simulink model "tire"  (R2020b)
settings: Solver=VariableStepAuto  StartTime=0.0  StopTime=10.0  RelTol=1e-3
InitFcn:
  | mdl = 'tire';
  | wks = get_param(mdl, 'ModelWorkspace');
  | 
  | % ---- FRONT TIRES ----
  | 
  | % Load data for front tires
  | vals_struct_front = load('lateral_data_lut_FRONT.mat');
  | load_y_front = vals_struct_front.load_y;
  | 
  | % Set data for FR tire
  | sa_x_FR = vals_struct_front.sa_x;
  | lateral_coeff_FR = vals_struct_front.lat_coeff;
  | aligning_torque_FR = vals_struct_front.aligning_torque;
  | 
  | % Set data for FL tire
  | sa_x_FL = -flip(sa_x_FR);
  | lateral_coeff_FL = -flipud(lateral_coeff_FR);
  | aligning_torque_FL = -flipud(aligning_torque_FR);
  | 
  | % Set front workspace vars to this data
  | assignin(wks, 'sa_x_FR', sa_x_FR);
  | assignin(wks, 'sa_x_FL', sa_x_FL);
  | assignin(wks, 'load_y_front', load_y_front);
  | assignin(wks, 'lateral_coeff_FR', lateral_coeff_FR);
  | assignin(wks, 'lateral_coeff_FL', lateral_coeff_FL);
  | assignin(wks, 'aligning_torque_FR', aligning_torque_FR);
  | assignin(wks, 'aligning_torque_FL', aligning_torque_FL);
  | 
  | % ---- REAR TIRES ----
  | 
  | % Load data for rear tires
  | vals_struct_rear = load('lateral_data_lut_REAR.mat');
  | load_y_rear = vals_struct_rear.load_y;
  | 
  | % Set data for RR tire
  | sa_x_RR = vals_struct_rear.sa_x;
  | lateral_coeff_RR = vals_struct_rear.lat_coeff;
  | aligning_torque_RR = vals_struct_rear.aligning_torque;
  | 
  | % Set data for RL tire
  | sa_x_RL = -flip(sa_x_RR);
  | lateral_coeff_RL = -flipud(lateral_coeff_RR);
  | aligning_torque_RL = -flipud(aligning_torque_RR);
  | 
  | % Set rear workspace vars to this data
  | assignin(wks, 'sa_x_RR', sa_x_RR);
  | assignin(wks, 'sa_x_RL', sa_x_RL);
  | assignin(wks, 'load_y_rear', load_y_rear);
  | assignin(wks, 'lateral_coeff_RR', lateral_coeff_RR);
  | assignin(wks, 'lateral_coeff_RL', lateral_coeff_RL);
  | assignin(wks, 'aligning_torque_RR', aligning_torque_RR);
  | assignin(wks, 'aligning_torque_RL', aligning_torque_RL);
model workspace (MAT data in the model file):
  aligning_torque = []
  aligning_torque_FL = [0.632054514609 1.00030929496 1.3564832949 1.69993473408 2.03003955804 2.34619584294 2.64782835053 2.93439319713 3.20538259517 3.4603296206 3.69881295493 3.92046154611 ... (18361 elements, 301x61)]
  aligning_torque_FR = [-8.27629240449 -7.94698029872 -7.63155523092 -7.33058213037 -7.04459380991 -6.7740862219 -6.51951369497 -6.28128420344 -6.05975472552 -5.85522675004 -5.66794199447 -5.49807839857 ... (18361 elements, 301x61)]
  aligning_torque_RL = [53.8378936848 52.3526089047 50.876903499 49.4110361793 47.9552665479 46.509854779 45.0750612888 43.6511464002 42.23837 40.836991194 39.4472679592 38.069456796 ... (18361 elements, 301x61)]
  aligning_torque_RR = [57.9779733339 55.1587439621 52.2420091829 49.2227619878 46.0969933513 42.8622156405 39.5181440804 36.0675717001 32.5174763364 28.8803985882 25.1761245506 21.4336928492 ... (18361 elements, 301x61)]
  lateral_coeff = []
  lateral_coeff_FL = [-2.62522245811 -2.64027696786 -2.65519252593 -2.6699687689 -2.68460531112 -2.69910174378 -2.71345763408 -2.72767252434 -2.74174593098 -2.75567734364 -2.76946622413 -2.7831120054 ... (18361 elements, 301x61)]
  lateral_coeff_FR = [-2.31568506961 -2.3309279537 -2.34603248296 -2.3609983259 -2.37582512996 -2.39051252072 -2.40506010102 -2.41946745011 -2.43373412279 -2.44785964843 -2.46184353006 -2.47568524338 ... (18361 elements, 301x61)]
  lateral_coeff_RL = [-2.38815959379 -2.39206360714 -2.39593787741 -2.39978203345 -2.40359569234 -2.407378459 -2.41112992576 -2.4148496719 -2.41853726322 -2.42219225158 -2.42581417433 -2.42940255388 ... (18361 elements, 301x61)]
  lateral_coeff_RR = [-2.49073654046 -2.49455737452 -2.49834746536 -2.50210640915 -2.50583378914 -2.50952917523 -2.51319212352 -2.51682217581 -2.52041885907 -2.52398168491 -2.52751014907 -2.53100373076 ... (18361 elements, 301x61)]
  load_y = []
  load_y_front = [0 -20 -40 -60 -80 -100 -120 -140 -160 -180 -200 -220 -240 -260 -280 -300 -320 -340 -360 -380 -400 -420 -440 -460 -480 -500 -520 -540 -560 -580 -600 -620 -640 -660 -680 -700 -720 -740 -760 -780 -800 -820 -840 -860 -880 -900 -920 -940 -960 -980 -1000 -1020 -1040 -1060 -1080 -1100 -1120 -1140 -1160 -1180 -1200]
  load_y_rear = [0 -20 -40 -60 -80 -100 -120 -140 -160 -180 -200 -220 -240 -260 -280 -300 -320 -340 -360 -380 -400 -420 -440 -460 -480 -500 -520 -540 -560 -580 -600 -620 -640 -660 -680 -700 -720 -740 -760 -780 -800 -820 -840 -860 -880 -900 -920 -940 -960 -980 -1000 -1020 -1040 -1060 -1080 -1100 -1120 -1140 -1160 -1180 -1200]
  sa_x = []
  sa_x_FL = [-0.261799387799 -0.260054058547 -0.258308729295 -0.256563400043 -0.254818070791 -0.253072741539 -0.251327412287 -0.249582083035 -0.247836753783 -0.246091424531 -0.244346095279 -0.242600766027 ... (301 elements, 1x301)]
  sa_x_FR = [-0.261799387799 -0.260054058547 -0.258308729295 -0.256563400043 -0.254818070791 -0.253072741539 -0.251327412287 -0.249582083035 -0.247836753783 -0.246091424531 -0.244346095279 -0.242600766027 ... (301 elements, 1x301)]
  sa_x_RL = [-0.261799387799 -0.260054058547 -0.258308729295 -0.256563400043 -0.254818070791 -0.253072741539 -0.251327412287 -0.249582083035 -0.247836753783 -0.246091424531 -0.244346095279 -0.242600766027 ... (301 elements, 1x301)]
  sa_x_RR = [-0.261799387799 -0.260054058547 -0.258308729295 -0.256563400043 -0.254818070791 -0.253072741539 -0.251327412287 -0.249582083035 -0.247836753783 -0.246091424531 -0.244346095279 -0.242600766027 ... (301 elements, 1x301)]
settings Model: ParameterArgumentNames=aligning_torque,lateral_coeff,load_y,sa_x  OrderedModelArguments=off  Creator=Matthew  LastModifiedBy=Matthew

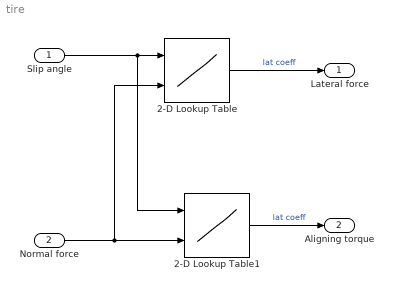
== system tire ==
  Slip angle : Inport
  Normal force : Inport  Port=2
  2-D Lookup Table : Lookup_n-D  BreakpointsForDimension1=sa_x  BreakpointsForDimension2=load_y  Table=lateral_coeff  InternalRulePriority=Speed  RndMeth=Simplest  InputSameDT=on
      settings: InputPortMap=u0,u1
  2-D Lookup Table1 : Lookup_n-D  BreakpointsForDimension1=sa_x  BreakpointsForDimension2=load_y  Table=aligning_torque  InternalRulePriority=Speed  RndMeth=Simplest  InputSameDT=on
      settings: InputPortMap=u0,u1
  Lateral force : Outport
  Aligning torque : Outport  Port=2
  wires:
  Slip angle/1 -> 2-D Lookup Table1/1, 2-D Lookup Table/1
  Normal force/1 -> 2-D Lookup Table/2, 2-D Lookup Table1/2
  2-D Lookup Table/1 -> Lateral force/1  "lat coeff"
  2-D Lookup Table1/1 -> Aligning torque/1  "lat coeff"
